simulink model "tesdd"  (R2012b)
(part 2 of 52)

      | %     current_names = textscan(strtrim(strrep(strrep(get_param(blk, 'names'), ']', ''), '[', '')), '%s');
      | %     current_names = current_names{1};
      | %     numios = length(current_names);
      | %     if length(current_types) ~= numios,
      | %         error('%d field names specified, but %d types?', numios, length(current_types));
      | %     end
      | % end
      | problem = 0;
      | for ctr = 1 : numios,
      |     t = current_types(ctr);
      |     if (t < 0) || (t > 2),
      |         problem = t;
      |         ctr = numios + 1;
      |     end
      | end
      | if problem ~= 0,
      |     error('Type cannot be %i, must be 0, 1 or 2.', problem);
      | end
      mask Callback bin_pts:
      | swreg_maskcheck(gcb);
      | % blk = gcb;
      | % mode = get_param(blk, 'mode');
      | % current_bins = eval(get_param(blk, 'bin_pts'));
      | % if (strcmp(mode, 'one value') || strcmp(mode, 'fields of equal size')) && (length(current_bins) > 1),
      | %     error('Only one binary pt may be specified for this mode.');
      | % elseif strcmp(mode, 'fields of arbitrary size')
      | %     current_names = textscan(strtrim(strrep(strrep(get_param(blk, 'names'), ']', ''), '[', '')), '%s');
      | %     current_names = current_names{1};
      | %     numios = length(current_names);
      | %     if length(current_bins) ~= numios,
      | %         error('%d field names specified, but %d binary pts?', numios, length(current_bins));
      | %     end
      | % end
  sw_timestamp2 : Subsystem  Tag=xps:sw_reg  AncestorBlock=xps_library/software register  mask(swreg){mode=one value, io_dir=From Processor, io_delay=0, sample_period=1, names=reg, bitwidths=32, arith_types=0, bin_pts=0, sim_port=on, show_format=off}
      mask prompts: io_dir "I/O direction"; io_delay "I/O delay"; sample_period "Sample period"; names "Name:"; bitwidths "Bitwidth:"; arith_types "Type (ufix=0, fix=1, bool=2):"; bin_pts "Binary pt:"; sim_port "Provide sim input/output?"; show_format "Print format string?"
      mask init:
      | swreg_init(gcb)
      settings: AttributesFormatString=1input
      mask TypeOptions mode: one value | fields of equal size | fields of arbitrary size
      mask Callback mode: swreg_cb(gcb);
      mask TypeOptions io_dir: To Processor | From Processor
      mask Callback io_dir:
      | mask_enables = get_param(gcb, 'MaskEnables');
      | mask_names = get_param(gcb, 'MaskNames');
      | if strcmp(get_param(gcb, 'io_dir'), 'To Processor'),
      |     mask_enables{ismember(mask_names, 'sample_period')} = 'off';
      | else
      |     mask_enables{ismember(mask_names, 'sample_period')} = 'on';
      | end
      | set_param(gcb, 'MaskEnables', mask_enables);
      mask Callback bitwidths:
      | swreg_maskcheck(gcb);
      | % blk = gcb;
      | % mode = get_param(blk, 'mode');
      | % current_widths = eval(get_param(blk, 'bitwidths'));
      | % if (strcmp(mode, 'one value') || strcmp(mode, 'fields of equal size')) && (length(current_widths) > 1),
      | %     error('Only one width may be specified for this mode.');
      | % elseif strcmp(mode, 'fields of arbitrary size')
      | %     current_names = textscan(strtrim(strrep(strrep(get_param(blk, 'names'), ']', ''), '[', '')), '%s');
      | %     current_names = current_names{1};
      | %     numios = length(current_names);
      | %     if length(current_widths) ~= numios,
      | %         error('%d field names specified, but %d widths?', numios, length(current_widths));
      | %     end
      | % end
      | % total_width = 0;
      | % for ctr = 1 : length(current_widths),
      | %     total_width = total_width + current_widths(ctr);
      | % end
      | % if total_width > 32,
      | %     error('Total width must be 32 or less, set to %d.', total_width);
      | % end
      mask Callback arith_types:
      | [numios, ~, ~, ~, current_types] = swreg_maskcheck(gcb);
      | % blk = gcb;
      | % mode = get_param(blk, 'mode');
      | % current_types = eval(get_param(blk, 'arith_types'));
      | % numios = length(current_types);
      | % if (strcmp(mode, 'one value') || strcmp(mode, 'fields of equal size')) && (length(current_types) > 1),
      | %     error('Only one type may be specified for this mode.');
      | % elseif strcmp(mode, 'fields of arbitrary size')
      | %     current_names = textscan(strtrim(strrep(strrep(get_param(blk, 'names'), ']', ''), '[', '')), '%s');
      | %     current_names = current_names{1};
      | %     numios = length(current_names);
      | %     if length(current_types) ~= numios,
      | %         error('%d field names specified, but %d types?', numios, length(current_types));
      | %     end
      | % end
      | problem = 0;
      | for ctr = 1 : numios,
      |     t = current_types(ctr);
      |     if (t < 0) || (t > 2),
      |         problem = t;
      |         ctr = numios + 1;
      |     end
      | end
      | if problem ~= 0,
      |     error('Type cannot be %i, must be 0, 1 or 2.', problem);
      | end
      mask Callback bin_pts:
      | swreg_maskcheck(gcb);
      | % blk = gcb;
      | % mode = get_param(blk, 'mode');
      | % current_bins = eval(get_param(blk, 'bin_pts'));
      | % if (strcmp(mode, 'one value') || strcmp(mode, 'fields of equal size')) && (length(current_bins) > 1),
      | %     error('Only one binary pt may be specified for this mode.');
      | % elseif strcmp(mode, 'fields of arbitrary size')
      | %     current_names = textscan(strtrim(strrep(strrep(get_param(blk, 'names'), ']', ''), '[', '')), '%s');
      | %     current_names = current_names{1};
      | %     numios = length(current_names);
      | %     if length(current_bins) ~= numios,
      | %         error('%d field names specified, but %d binary pts?', numios, length(current_bins));
      | %     end
      | % end
  syncDelay : Subsystem  Tag=xps:sw_reg  AncestorBlock=xps_library/software register  mask(swreg){mode=one value, io_dir=From Processor, io_delay=0, sample_period=1, names=reg, bitwidths=16, arith_types=0, bin_pts=0, sim_port=on, show_format=off}
      mask prompts: io_dir "I/O direction"; io_delay "I/O delay"; sample_period "Sample period"; names "Name:"; bitwidths "Bitwidth:"; arith_types "Type (ufix=0, fix=1, bool=2):"; bin_pts "Binary pt:"; sim_port "Provide sim input/output?"; show_format "Print format string?"
      mask init:
      | swreg_init(gcb)
      settings: AttributesFormatString=1input
      mask TypeOptions mode: one value | fields of equal size | fields of arbitrary size
      mask Callback mode: swreg_cb(gcb);
      mask TypeOptions io_dir: To Processor | From Processor
      mask Callback io_dir:
      | mask_enables = get_param(gcb, 'MaskEnables');
      | mask_names = get_param(gcb, 'MaskNames');
      | if strcmp(get_param(gcb, 'io_dir'), 'To Processor'),
      |     mask_enables{ismember(mask_names, 'sample_period')} = 'off';
      | else
      |     mask_enables{ismember(mask_names, 'sample_period')} = 'on';
      | end
      | set_param(gcb, 'MaskEnables', mask_enables);
      mask Callback bitwidths:
      | swreg_maskcheck(gcb);
      | % blk = gcb;
      | % mode = get_param(blk, 'mode');
      | % current_widths = eval(get_param(blk, 'bitwidths'));
      | % if (strcmp(mode, 'one value') || strcmp(mode, 'fields of equal size')) && (length(current_widths) > 1),
      | %     error('Only one width may be specified for this mode.');
      | % elseif strcmp(mode, 'fields of arbitrary size')
      | %     current_names = textscan(strtrim(strrep(strrep(get_param(blk, 'names'), ']', ''), '[', '')), '%s');
      | %     current_names = current_names{1};
      | %     numios = length(current_names);
      | %     if length(current_widths) ~= numios,
      | %         error('%d field names specified, but %d widths?', numios, length(current_widths));
      | %     end
      | % end
      | % total_width = 0;
      | % for ctr = 1 : length(current_widths),
      | %     total_width = total_width + current_widths(ctr);
      | % end
      | % if total_width > 32,
      | %     error('Total width must be 32 or less, set to %d.', total_width);
      | % end
      mask Callback arith_types:
      | [numios, ~, ~, ~, current_types] = swreg_maskcheck(gcb);
      | % blk = gcb;
      | % mode = get_param(blk, 'mode');
      | % current_types = eval(get_param(blk, 'arith_types'));
      | % numios = length(current_types);
      | % if (strcmp(mode, 'one value') || strcmp(mode, 'fields of equal size')) && (length(current_types) > 1),
      | %     error('Only one type may be specified for this mode.');
      | % elseif strcmp(mode, 'fields of arbitrary size')
      | %     current_names = textscan(strtrim(strrep(strrep(get_param(blk, 'names'), ']', ''), '[', '')), '%s');
      | %     current_names = current_names{1};
      | %     numios = length(current_names);
      | %     if length(current_types) ~= numios,
      | %         error('%d field names specified, but %d types?', numios, length(current_types));
      | %     end
      | % end
      | problem = 0;
      | for ctr = 1 : numios,
      |     t = current_types(ctr);
      |     if (t < 0) || (t > 2),
      |         problem = t;
      |         ctr = numios + 1;
      |     end
      | end
      | if problem ~= 0,
      |     error('Type cannot be %i, must be 0, 1 or 2.', problem);
      | end
      mask Callback bin_pts:
      | swreg_maskcheck(gcb);
      | % blk = gcb;
      | % mode = get_param(blk, 'mode');
      | % current_bins = eval(get_param(blk, 'bin_pts'));
      | % if (strcmp(mode, 'one value') || strcmp(mode, 'fields of equal size')) && (length(current_bins) > 1),
      | %     error('Only one binary pt may be specified for this mode.');
      | % elseif strcmp(mode, 'fields of arbitrary size')
      | %     current_names = textscan(strtrim(strrep(strrep(get_param(blk, 'names'), ']', ''), '[', '')), '%s');
      | %     current_names = current_names{1};
      | %     numios = length(current_names);
      | %     if length(current_bins) ~= numios,
      | %         error('%d field names specified, but %d binary pts?', numios, length(current_bins));
      | %     end
      | % end
  sync_bit1 : xbsIndex_r4/Slice  nbits=1  boolean_output=on  mode=Upper Bit Location + Width  bit1=-2  base1=MSB of Input  bit0=0  base0=LSB of Input  dbl_ovrd=off  block_type=slice
  sync_bit7 : xbsIndex_r4/Slice  nbits=1  boolean_output=on  mode=Upper Bit Location + Width  bit1=-2  base1=MSB of Input  bit0=0  base0=LSB of Input  dbl_ovrd=off  block_type=slice
  sync_in : xps_library/gpio  Tag=xps:gpio  io_group=ROACH2:sync_in  io_dir=in  arith_type=Boolean  bitwidth=1  bin_pt=0  bit_index=0  sample_period=1  use_single_ended=off  use_ddr=off  reg_iob=on  reg_clk_phase=0  termination=None
  sync_out : xps_library/gpio  Tag=xps:gpio  io_group=ROACH2:sync_out  io_dir=out  arith_type=Boolean  bitwidth=1  bin_pt=0  bit_index=0  sample_period=1  use_single_ended=off  use_ddr=off  reg_iob=on  reg_clk_phase=0  termination=None
  top16_{1..8} (8 alike) : xbsIndex_r4/Slice  nbits=16  boolean_output=off  mode=Upper Bit Location + Width  bit1=0  base1=MSB of Input  bit0=0  base0=MSB of Input  dbl_ovrd=off  block_type=slice
  txdestip : Subsystem  Tag=xps:sw_reg  AncestorBlock=xps_library/software register  mask(swreg){mode=one value, io_dir=From Processor, io_delay=0, sample_period=1, names=reg, bitwidths=32, arith_types=0, bin_pts=0, sim_port=on, show_format=off}
      mask prompts: io_dir "I/O direction"; io_delay "I/O delay"; sample_period "Sample period"; names "Name:"; bitwidths "Bitwidth:"; arith_types "Type (ufix=0, fix=1, bool=2):"; bin_pts "Binary pt:"; sim_port "Provide sim input/output?"; show_format "Print format string?"
      mask init:
      | swreg_init(gcb)
      settings: AttributesFormatString=1input
      mask TypeOptions mode: one value | fields of equal size | fields of arbitrary size
      mask Callback mode: swreg_cb(gcb);
      mask TypeOptions io_dir: To Processor | From Processor
      mask Callback io_dir:
      | mask_enables = get_param(gcb, 'MaskEnables');
      | mask_names = get_param(gcb, 'MaskNames');
      | if strcmp(get_param(gcb, 'io_dir'), 'To Processor'),
      |     mask_enables{ismember(mask_names, 'sample_period')} = 'off';
      | else
      |     mask_enables{ismember(mask_names, 'sample_period')} = 'on';
      | end
      | set_param(gcb, 'MaskEnables', mask_enables);
      mask Callback bitwidths:
      | swreg_maskcheck(gcb);
      | % blk = gcb;
      | % mode = get_param(blk, 'mode');
      | % current_widths = eval(get_param(blk, 'bitwidths'));
      | % if (strcmp(mode, 'one value') || strcmp(mode, 'fields of equal size')) && (length(current_widths) > 1),
      | %     error('Only one width may be specified for this mode.');
      | % elseif strcmp(mode, 'fields of arbitrary size')
      | %     current_names = textscan(strtrim(strrep(strrep(get_param(blk, 'names'), ']', ''), '[', '')), '%s');
      | %     current_names = current_names{1};
      | %     numios = length(current_names);
      | %     if length(current_widths) ~= numios,
      | %         error('%d field names specified, but %d widths?', numios, length(current_widths));
      | %     end
      | % end
      | % total_width = 0;
      | % for ctr = 1 : length(current_widths),
      | %     total_width = total_width + current_widths(ctr);
      | % end
      | % if total_width > 32,
      | %     error('Total width must be 32 or less, set to %d.', total_width);
      | % end
      mask Callback arith_types:
      | [numios, ~, ~, ~, current_types] = swreg_maskcheck(gcb);
      | % blk = gcb;
      | % mode = get_param(blk, 'mode');
      | % current_types = eval(get_param(blk, 'arith_types'));
      | % numios = length(current_types);
      | % if (strcmp(mode, 'one value') || strcmp(mode, 'fields of equal size')) && (length(current_types) > 1),
      | %     error('Only one type may be specified for this mode.');
      | % elseif strcmp(mode, 'fields of arbitrary size')
      | %     current_names = textscan(strtrim(strrep(strrep(get_param(blk, 'names'), ']', ''), '[', '')), '%s');
      | %     current_names = current_names{1};
      | %     numios = length(current_names);
      | %     if length(current_types) ~= numios,
      | %         error('%d field names specified, but %d types?', numios, length(current_types));
      | %     end
      | % end
      | problem = 0;
      | for ctr = 1 : numios,
      |     t = current_types(ctr);
      |     if (t < 0) || (t > 2),
      |         problem = t;
      |         ctr = numios + 1;
      |     end
      | end
      | if problem ~= 0,
      |     error('Type cannot be %i, must be 0, 1 or 2.', problem);
      | end
      mask Callback bin_pts:
      | swreg_maskcheck(gcb);
      | % blk = gcb;
      | % mode = get_param(blk, 'mode');
      | % current_bins = eval(get_param(blk, 'bin_pts'));
      | % if (strcmp(mode, 'one value') || strcmp(mode, 'fields of equal size')) && (length(current_bins) > 1),
      | %     error('Only one binary pt may be specified for this mode.');
      | % elseif strcmp(mode, 'fields of arbitrary size')
      | %     current_names = textscan(strtrim(strrep(strrep(get_param(blk, 'names'), ']', ''), '[', '')), '%s');
      | %     current_names = current_names{1};
      | %     numios = length(current_names);
      | %     if length(current_bins) ~= numios,
      | %         error('%d field names specified, but %d binary pts?', numios, length(current_bins));
      | %     end
      | % end
  txdestport : Subsystem  Tag=xps:sw_reg  AncestorBlock=xps_library/software register  mask(swreg){mode=one value, io_dir=From Processor, io_delay=0, sample_period=1, names=reg, bitwidths=16, arith_types=0, bin_pts=0, sim_port=on, show_format=off}
      mask prompts: io_dir "I/O direction"; io_delay "I/O delay"; sample_period "Sample period"; names "Name:"; bitwidths "Bitwidth:"; arith_types "Type (ufix=0, fix=1, bool=2):"; bin_pts "Binary pt:"; sim_port "Provide sim input/output?"; show_format "Print format string?"
      mask init:
      | swreg_init(gcb)
      settings: AttributesFormatString=1input
      mask TypeOptions mode: one value | fields of equal size | fields of arbitrary size
      mask Callback mode: swreg_cb(gcb);
      mask TypeOptions io_dir: To Processor | From Processor
      mask Callback io_dir:
      | mask_enables = get_param(gcb, 'MaskEnables');
      | mask_names = get_param(gcb, 'MaskNames');
      | if strcmp(get_param(gcb, 'io_dir'), 'To Processor'),
      |     mask_enables{ismember(mask_names, 'sample_period')} = 'off';
      | else
      |     mask_enables{ismember(mask_names, 'sample_period')} = 'on';
      | end
      | set_param(gcb, 'MaskEnables', mask_enables);
      mask Callback bitwidths:
      | swreg_maskcheck(gcb);
      | % blk = gcb;
      | % mode = get_param(blk, 'mode');
      | % current_widths = eval(get_param(blk, 'bitwidths'));
      | % if (strcmp(mode, 'one value') || strcmp(mode, 'fields of equal size')) && (length(current_widths) > 1),
      | %     error('Only one width may be specified for this mode.');
      | % elseif strcmp(mode, 'fields of arbitrary size')
      | %     current_names = textscan(strtrim(strrep(strrep(get_param(blk, 'names'), ']', ''), '[', '')), '%s');
      | %     current_names = current_names{1};
      | %     numios = length(current_names);
      | %     if length(current_widths) ~= numios,
      | %         error('%d field names specified, but %d widths?', numios, length(current_widths));
      | %     end
      | % end
      | % total_width = 0;
      | % for ctr = 1 : length(current_widths),
      | %     total_width = total_width + current_widths(ctr);
      | % end
      | % if total_width > 32,
      | %     error('Total width must be 32 or less, set to %d.', total_width);
      | % end
      mask Callback arith_types:
      | [numios, ~, ~, ~, current_types] = swreg_maskcheck(gcb);
      | % blk = gcb;
      | % mode = get_param(blk, 'mode');
      | % current_types = eval(get_param(blk, 'arith_types'));
      | % numios = length(current_types);
      | % if (strcmp(mode, 'one value') || strcmp(mode, 'fields of equal size')) && (length(current_types) > 1),
      | %     error('Only one type may be specified for this mode.');
      | % elseif strcmp(mode, 'fields of arbitrary size')
      | %     current_names = textscan(strtrim(strrep(strrep(get_param(blk, 'names'), ']', ''), '[', '')), '%s');
      | %     current_names = current_names{1};
      | %     numios = length(current_names);
      | %     if length(current_types) ~= numios,
      | %         error('%d field names specified, but %d types?', numios, length(current_types));
      | %     end
      | % end
      | problem = 0;
      | for ctr = 1 : numios,
      |     t = current_types(ctr);
      |     if (t < 0) || (t > 2),
      |         problem = t;
      |         ctr = numios + 1;
      |     end
      | end
      | if problem ~= 0,
      |     error('Type cannot be %i, must be 0, 1 or 2.', problem);
      | end
      mask Callback bin_pts:
      | swreg_maskcheck(gcb);
      | % blk = gcb;
      | % mode = get_param(blk, 'mode');
      | % current_bins = eval(get_param(blk, 'bin_pts'));
      | % if (strcmp(mode, 'one value') || strcmp(mode, 'fields of equal size')) && (length(current_bins) > 1),
      | %     error('Only one binary pt may be specified for this mode.');
      | % elseif strcmp(mode, 'fields of arbitrary size')
      | %     current_names = textscan(strtrim(strrep(strrep(get_param(blk, 'names'), ']', ''), '[', '')), '%s');
      | %     current_names = current_names{1};
      | %     numios = length(current_names);
      | %     if length(current_bins) ~= numios,
      | %         error('%d field names specified, but %d binary pts?', numios, length(current_bins));
      | %     end
      | % end
  zero_bool_{1..4} (4 alike) : xbsIndex_r4/Constant  const=1  gui_display_data_type=Boolean  arith_type=Boolean  n_bits=36  bin_pt=0  preci_type=Single  exp_width=8  frac_width=24  explicit_period=on  period=1  equ=P=C  opselect=C  inp2=PCIN>>17  opr=+  inp1=P  carry=CIN  dbl_ovrd=off  block_type=constant
  zero_bool_7 : xbsIndex_r4/Constant  const=0  gui_display_data_type=Boolean  arith_type=Boolean  n_bits=36  bin_pt=0  preci_type=Single  exp_width=8  frac_width=24  explicit_period=on  period=1  equ=P=C  opselect=C  inp2=PCIN>>17  opr=+  inp1=P  carry=CIN  dbl_ovrd=off  block_type=constant
  wires:
  SRAM_LUT/9(syncout) -> Delay30/1
  MKID_ADC/9(sync) -> Delay29/1
  bool/1 -> octoscope/11(tr2), octoscope/12(tr3), octoscope/16(we3), octoscope/13(we0), octoscope/15(we2), octoscope/14(we1)
  SRAM_LUT/10(bus128) -> Delay36/1, Delay8/1
  Delay25/1 -> WindowAndFFT/6(In6), octoscope/5(in5)
  Delay21/1 -> WindowAndFFT/4(In4), octoscope/1(In1)
  Delay22/1 -> WindowAndFFT/5(In5), octoscope/2(In2)
  Delay26/1 -> octoscope/6(in6), WindowAndFFT/8(In8)
  Delay23/1 -> octoscope/3(In3), WindowAndFFT/7(In7)
  Delay27/1 -> WindowAndFFT/9(In9), octoscope/7(in7)
  Delay24/1 -> octoscope/4(In4), WindowAndFFT/11(In11)
  Delay28/1 -> WindowAndFFT/10(In10), octoscope/8(in8)
  zero_bool_3/1 -> FIFO64_4/7, FIFO64_4/8
  FIFO64_4/8 -> Delay59/1
  [rdchan_a] -> FIFO64_4/4
  fifoRdSettingsA/1(Out1) -> [dumpfifo]
  fifoRdSettingsA/3(Out3) -> [wrrawdata]
  fifoRdSettingsA/4(Out4) -> [is_look_sync]
  fifoRdSettingsA/5(Out5) -> [flushfifo]
  Constant/1 -> lastReadChanA/1(sim_1)
  fifoRdSettingsA/6(Out6) -> [fiforst]
  [fiforst] -> FIFO64_4/6
  [fiford1] -> FIFO64_4/5
  extract_sync_enable_2/2(cmplx_dout) -> dataformatter2/3(data)
  [rdchan_b] -> FIFO64_2/4
  [fiford2] -> FIFO64_2/5
  [fiforst] -> FIFO64_2/6
  FIFO64_2/1 -> extract_sync_enable_2/2(cmplx_din)
  FIFO64_2/8 -> Delay20/1
  fftcoefselector/11(fftfoecsync) -> Delay35/1, [fft_coef_sync]
  zero_bool_7/1 -> octoscope1/15(we2), octoscope1/14(we1), octoscope1/13(we0), octoscope1/12(tr3), octoscope1/10(tr1), octoscope1/11(tr2), octoscope1/16(we3)
  fifoRdSettingsA/7(Out7) -> [drop_all_events]
  fifoRdSettingsA/8(Out8) -> [ethernet_rst]
  [fiforst] -> FIFO64_1/6
  [fiforst] -> FIFO64_3/6
  [dumpfifo] -> MCode2/1
  FIFO64_3/2 -> MCode2/2
  FIFO64_3/5 -> MCode2/3
  FIFO64_3/8 -> Delay6/1
  [rdchan_b] -> FIFO64_3/4
  [rdchan_a] -> FIFO64_1/4
  [fiford1] -> FIFO64_1/5
  [fiford2] -> FIFO64_3/5
  dataformatter1/1(dout) -> Delay15/1
  Delay8/1 -> MKID_DAC/1(buss128)
  Delay29/1 -> octoscope/9(tr0)
  Delay30/1 -> fftcoefselector/2(lut_sync), octoscope/10(tr1)
  fifoRdSettingsA/9(Out9) -> [rst_full_counters]
  Counter3/1 -> fifowriB/1(out_reg)
  [rst_full_counters] -> Counter3/1
  Counter4/1 -> fifowrC/1(out_reg)
  [rst_full_counters] -> Counter4/1
  Counter5/1 -> fifowrD/1(out_reg)
  [rst_full_counters] -> Counter21/1
  Counter7/1 -> evtfifowrB/1(out_reg)
  [rst_full_counters] -> Counter7/1
  Counter9/1 -> outfifowrB/1(out_reg)
  [rst_full_counters] -> Counter9/1
  [datapath_enableb] -> extract_sync_enable_2/4(en)
  Delay20/1 -> extract_sync_enable_2/1(dvld_in)
  [datapath_enableb] -> extract_sync_enable_1/4(en)
  extract_sync_enable_1/2(cmplx_dout) -> dataformatter1/3(data)
  c_to_ri3/1 -> top16_8/1
  c_to_ri4/1 -> top16_2/1
  c_to_ri1/1 -> top16_3/1
  c_to_ri3/2 -> top16_5/1
  c_to_ri4/2 -> top16_6/1
  c_to_ri1/2 -> top16_7/1
  Delay35/1 -> octoscope1/9(tr0)
  Delay31/1 -> c_to_ri2/1
  Delay32/1 -> c_to_ri3/1
  Delay33/1 -> c_to_ri4/1
  Delay34/1 -> c_to_ri1/1
  top16_2/1 -> octoscope1/3(In3)
  top16_3/1 -> octoscope1/4(In4)
  top16_4/1 -> octoscope1/5(in5)
  top16_5/1 -> octoscope1/6(in6)
  top16_6/1 -> octoscope1/7(in7)
  top16_7/1 -> octoscope1/8(in8)
  Delay36/1 -> MKID_ADC/1(in128)
  fftcoefselector/13(topfbsyncin) -> WindowAndFFT/2(In2), [start_fft_sync]
  c_to_ri2/1 -> top16_1/1
  c_to_ri2/2 -> top16_4/1
  top16_1/1 -> octoscope1/1(In1)
  top16_8/1 -> octoscope1/2(In2)
  Concat/1 -> FIFO64_3/3
  Concat4/1 -> FIFO64_1/3
  Concat2/1 -> FIFO64_2/3
  Concat3/1 -> FIFO64_4/3
  [is_look_sync] -> dataformatter1/4(is_pulse)
  [is_look_sync] -> dataformatter2/4(is_pulse)
  Constant5/1 -> syncDelay/1(sim_1)
  Pulse Generator/1 -> sync_in/1
  fifoRdSettingsA/2(Out2) -> [fsmrst]
  lastReadChanA/1(in_reg) -> Delay3/1
  Constant6/1 -> readFifoSize/1(sim_1)
  [fsmrst] -> MCode2/4
  MCode2/3 -> lsb0_5_1/1, [current_chan2]
  MCode2/5 -> [datapath_enableb]
  extract_sync_enable_1/1(dvld_out) -> MCode2/5
  [flushfifo] -> MCode2/8
  [is_look_sync] -> MCode2/11
  bool_5/1 -> MCode2/7
  bool_6/1 -> MCode2/12
  sync_bit1/1 -> Delay43/1
  Delay43/1 -> MCode2/10
  dataformatter2/1(dout) -> Delay/1
  sync_in/1 -> Delay13/1
  fifoRdSettingsA/10(Out10) -> [sync_source]
  [sync_source] -> Mux/1
  RampGenerator/1(ramp) -> SigmaDeltaSecOrder/1(DataIn)
  RampGenerator/2(syncout) -> Mux/3
  Constant2/1 -> sw_timestamp2/1(sim_1)
  fftcoefselector/17(timestamp) -> [fftcounter]
  extract_sync_enable_2/4(swts) -> [swtimestamp2bit_1]
  sw_timestamp/1(in_reg) -> Delay1/1
  FIFO64_3/1 -> sync_bit1/1, extract_sync_enable_1/2(cmplx_din)
  Counter14/1 -> numdoneevts1/1(out_reg)
  [rst_full_counters] -> Counter14/1
  Counter19/1 -> evtfifordB/1(out_reg)
  [rst_full_counters] -> Counter19/1
  Constant3/1 -> sw_timestamp/1(sim_1)
  SigmaDeltaSecOrder/1(DataOut) -> Delay4/1
  Delay4/1 -> Delay12/1
  fifoRdSettingsA/11(Out11) -> [en_ramp_gen]
  [en_ramp_gen] -> Delay4/2
  MCode2/6 -> [wr_data_sel2]
  MCode2/2 -> [wr_big_fifo2], Counter7/2
  fifoRdSettingsA/12(Out12) -> [fluxdemod]
  fifoRdSettingsA/13(Out13) -> [savefluxraw]
  [fsmrst] -> Delay38/1
  [flushfifo] -> Delay39/1
  FRD1/1(evt_fifo_rd) -> datacombine/8(rddata), Counter19/2
  [fluxdemod] -> Delay40/1
  [savefluxraw] -> Delay42/1
  FRD1/3(out_wr) -> Delay46/1, Counter9/2
  Counter20/1 -> chanFifoFull2/1(out_reg)
  FIFO64_1/6 -> Counter20/2
  [rst_full_counters] -> Counter20/1
  Counter21/1 -> chanFifoFull3/1(out_reg)
  FIFO64_3/6 -> Counter21/2
  [savetranslated] -> Delay41/1
  RampTimingNew/1(synctofft) -> [syncsave]
  [rst_full_counters] -> RampTimingNew/1(rstcnt)
  sw_timestamp2/1(in_reg) -> Delay7/1
  [fft_coef_sync] -> RampTimingNew/3(fftcoefsync)
  syncDelay/1(in_reg) -> Delay9/1
  Mux/1 -> edge_detect/1(in), RampTimingNew/5(sync)
  RampTimingNew/2(numsync1) -> Delay10/1
  RampTimingNew/3(numsync) -> Delay11/1
  fftcoefselector/12(fftshiftx) -> WindowAndFFT/1(In1)
  fftcoefselector/15(stopfft) -> WindowAndFFT/3(In3)
  WindowAndFFT/2(fft2dly) -> FM/9(fft2dky), Delay31/1
  WindowAndFFT/4(fft2) -> FM/11(fft2), Delay33/1
  WindowAndFFT/5(fft3) -> FM/12(fft3), Delay34/1
  WindowAndFFT/1(Out5) -> fftcoefselector/1(fftsyncout)
  WindowAndFFT/3(fft3dly) -> FM/10(fft3dly), Delay32/1
  FM/9(dvldout4) -> FIFO64_3/2, Counter5/2
  FM/12(dout4) -> Concat/2
  FM/10(dout3) -> Concat4/2
  FM/6(dout2) -> Concat2/2
  FM/3(dout1) -> Concat3/2
  fftcoefselector/4(we2) -> FM/1(ff2d_dval), FM/3(f2_dval)
  fftcoefselector/5(we3) -> FM/2(f3d_dval), FM/4(f3dval)
  fftcoefselector/8(chan2) -> FM/5(f2dchan), FM/7(f2chan)
  fftcoefselector/9(chan3) -> FM/6(f3dchan), FM/8(f3chan)
  [start_fft_sync] -> FM/13(rstaccum)
  FM/8(chanout3) -> FIFO64_1/1
  FM/11(chanout4) -> FIFO64_3/1
  FIFO64_2/4 -> Terminator5/1
  FIFO64_2/5 -> Terminator6/1
  FIFO64_2/6 -> Terminator7/1
  FIFO64_2/7 -> Terminator8/1
  FIFO64_2/9 -> Terminator9/1
  FIFO64_4/4 -> Terminator/1
  FIFO64_4/5 -> Terminator1/1
  FIFO64_4/6 -> Terminator2/1
  FIFO64_4/7 -> Terminator3/1
  FIFO64_4/9 -> Terminator4/1
  zero_bool_1/1 -> FIFO64_2/8, FIFO64_2/7
  zero_bool_2/1 -> FIFO64_1/8, FIFO64_1/7
  zero_bool_4/1 -> FIFO64_3/7, FIFO64_3/8
  Counter2/1 -> fifowrA/1(out_reg)
  fifoRdSettingsA/14(Out14) -> [savetranslated]
  [rst_full_counters] -> Counter2/1
  [syncsave] -> Concat/1
  [syncsave] -> Concat4/1
  [syncsave] -> Concat2/1
  [syncsave] -> Concat3/1
  [rst_full_counters] -> Counter5/1
  [event_length] -> MCode2/9
  readFifoSize/1(in_reg) -> Delay2/1
  [last_channel] -> MCode2/6
  [current_chan2] -> extract_sync_enable_2/3(chan)
  [current_chan2] -> dataformatter2/2(channel_)
  [wr_big_fifo2] -> Delay14/1
  [wr_data_sel2] -> dataformatter2/5(wr_data_sel)
  [swtimestamp32] -> dataformatter2/1(timestamp32_)
  [swtimestamp32] -> dataformatter1/1(timestamp32_)
  [current_chan2] -> extract_sync_enable_1/3(chan)
  [current_chan2] -> dataformatter1/2(channel_)
  MCode2/1 -> [fiford2]
  [wr_data_sel2] -> dataformatter1/5(wr_data_sel)
  [wr_big_fifo2] -> Delay16/1
  [ethernet_rst] -> Delay48/1
  [fsmrst] -> Delay49/1
  [flushfifo] -> Delay50/1
  txdestip/1(in_reg) -> Delay51/1
  txdestport/1(in_reg) -> Delay52/1
  [rst_full_counters] -> Delay47/1
  FRD1/2(dataout) -> Delay45/1
  GBEthernet/1(numtxeof) -> gbeofcount/1(out_reg)
  GBEthernet/3(numtxovf) -> gbtxovfcnt/1(out_reg)
  GBEthernet/6(numtxvld) -> gbdatalen/1(out_reg)
  GBEthernet/7(numfiford) -> outfifordA/1(out_reg)
  GBEthernet/10(numrd2) -> outfifordB/1(out_reg)
  Constant1/1 -> txdestport/1(sim_1), txdestip/1(sim_1)
  [event_length] -> Delay44/1
  MultByTwoUI8_/1(Out1) -> FRD1/1(evtlen)
  [event_length] -> Delay17/1
  datacombine/1(evt_fifo_rd) -> SinglaEvtFIFO1/3, SinglaEvtFIFO2/3
  [flushfifo] -> Delay18/1
  [fsmrst] -> Delay19/1
  [save_event2] -> Delay37/1
  SinglaEvtFIFO2/1 -> datacombine/3(data_in)
  SinglaEvtFIFO2/2 -> datacombine/2(fifo_empty)
  datacombine/3(dataout) -> FRD1/3(data_in)
  datacombine/4(empty) -> FRD1/2(fifo_empty)
  datacombine/2(evtdone) -> FRD1/4(new_evt_rdy)
  SinglaEvtFIFO1/1 -> datacombine/7(datain2)
  FM/7(dvldout3) -> FIFO64_1/2, Counter4/2
  MCode2/7 -> [save_event2], Counter14/2
  FM/2(dvalout1) -> FIFO64_4/2, Counter2/2
  FM/1(chanout1) -> FIFO64_4/1
  FM/4(chanout2) -> FIFO64_2/1
  FM/5(dvalout2) -> Counter3/2, FIFO64_2/2
  Delay1/1 -> [swtimestamp32]
  Delay2/1 -> [event_length]
  Delay3/1 -> [last_channel]
  Delay7/1 -> RampTimingNew/2(swts2)
  Delay9/1 -> RampTimingNew/4(syncdelay)
  Delay10/1 -> numSyncPulses1/1(out_reg)
  Delay11/1 -> numSyncPulses/1(out_reg)
  Delay12/1 -> sync_out/1
  Delay13/1 -> Mux/2
  MKID_ADC/1(i0) -> Delay21/1
  MKID_ADC/2(i1) -> Delay22/1
  MKID_ADC/3(i2) -> Delay23/1
  MKID_ADC/4(i3) -> Delay24/1
  MKID_ADC/5(q0) -> Delay25/1
  MKID_ADC/6(q1) -> Delay26/1
  MKID_ADC/7(q2) -> Delay27/1
  MKID_ADC/8(q3) -> Delay28/1
  Delay/1 -> SinglaEvtFIFO1/1
  Delay14/1 -> SinglaEvtFIFO1/2
  Delay15/1 -> SinglaEvtFIFO2/1
  Delay16/1 -> SinglaEvtFIFO2/2
  Delay17/1 -> datacombine/1(evtlen)
  Delay18/1 -> datacombine/6(clr_fifos)
  Delay19/1 -> datacombine/5(rst)
  Delay37/1 -> datacombine/4(new_evt_rdy)
  Delay38/1 -> FRD1/5(rst)
  Delay39/1 -> FRD1/6(clr_fifos)
  Delay40/1 -> FRD1/7(isflux_demod)
  Delay41/1 -> FRD1/9(circletrans)
  Delay42/1 -> FRD1/8(savefluxraw)
  Delay44/1 -> MultByTwoUI8_/1(In1)
  Delay45/1 -> GBEthernet/9(din2)
  Delay46/1 -> GBEthernet/10(wr2)
  Delay47/1 -> GBEthernet/8(rst)
  Delay48/1 -> GBEthernet/1(rstgbe)
  Delay49/1 -> GBEthernet/2(rstfsm)
  Delay50/1 -> GBEthernet/3(clrfifo)
  Delay51/1 -> GBEthernet/4(destip)
  Delay52/1 -> GBEthernet/5(destport)
  edge_detect/1(out) -> [rampsyncedge]
  [rampsyncedge] -> fftcoefselector/3(rampsync)
  [rst_full_counters] -> Counter1/1
  Counter1/1 -> SEFull/1(out_reg)
  SinglaEvtFIFO1/3 -> Counter1/2
  [rst_full_counters] -> Counter6/1
  Counter6/1 -> SEFull1/1(out_reg)
  SinglaEvtFIFO2/3 -> Counter6/2
  [rst_full_counters] -> datacombine/9(rstfull)
  Counter8/1 -> gbfull1/1(out_reg)
  [rst_full_counters] -> Counter10/1, Counter8/1
  GBEthernet/5(full1) -> Counter8/2
  Counter10/1 -> gbfull2/1(out_reg)
  GBEthernet/9(full2) -> Counter10/2
  [rst_full_counters] -> FRD1/10(rstfull)
  Delay6/1 -> extract_sync_enable_1/1(dvld_in)
  extract_sync_enable_4/2(cmplx_dout) -> dataformatter4/3(data)
  [dumpfifo] -> MCode1/1
  dataformatter3/1(dout) -> Delay54/1
  Counter16/1 -> evtfifowrB1/1(out_reg)
  [rst_full_counters] -> Counter16/1
  Counter17/1 -> outfifowrB1/1(out_reg)
  [rst_full_counters] -> Counter17/1
  [datapath_enablea] -> extract_sync_enable_4/4(en)
  Delay59/1 -> extract_sync_enable_4/1(dvld_in)
  [datapath_enablea] -> extract_sync_enable_3/4(en)
  extract_sync_enable_3/2(cmplx_dout) -> dataformatter3/3(data)
  [is_look_sync] -> dataformatter3/4(is_pulse)
  [is_look_sync] -> dataformatter4/4(is_pulse)
  [fsmrst] -> MCode1/4
  MCode1/3 -> lsb0_5_2/1, [current_chan1]
  MCode1/5 -> [datapath_enablea]
  extract_sync_enable_3/1(dvld_out) -> MCode1/5
  [flushfifo] -> MCode1/8
  [is_look_sync] -> MCode1/11
  bool_2/1 -> MCode1/7
  bool_3/1 -> MCode1/12
  sync_bit7/1 -> Delay66/1
  Delay66/1 -> MCode1/10
  dataformatter4/1(dout) -> Delay5/1
  extract_sync_enable_4/4(swts) -> [swtimestamp2bit_2]
  FIFO64_1/1 -> extract_sync_enable_3/2(cmplx_din), sync_bit7/1
  Counter12/1 -> numdoneevts2/1(out_reg)
  [rst_full_counters] -> Counter12/1
  Counter13/1 -> evtfifordB1/1(out_reg)
  [rst_full_counters] -> Counter13/1
  MCode1/6 -> [wr_data_sel1]
  MCode1/2 -> [wr_big_fifo1], Counter16/2
  [fsmrst] -> Delay61/1
  [flushfifo] -> Delay62/1
  FRD2/1(evt_fifo_rd) -> datacombine1/8(rddata), Counter13/2
  [fluxdemod] -> Delay63/1
  [savefluxraw] -> Delay65/1
  FRD2/3(out_wr) -> Delay69/1, Counter17/2
  [savetranslated] -> Delay64/1
  [event_length] -> MCode1/9
  [last_channel] -> MCode1/6
  [current_chan1] -> extract_sync_enable_4/3(chan)
  [current_chan1] -> dataformatter4/2(channel_)
  [wr_big_fifo1] -> Delay53/1
  [wr_data_sel1] -> dataformatter4/5(wr_data_sel)
  [swtimestamp32] -> dataformatter4/1(timestamp32_)
  [swtimestamp32] -> dataformatter3/1(timestamp32_)
  [current_chan1] -> extract_sync_enable_3/3(chan)
  [current_chan1] -> dataformatter3/2(channel_)
  MCode1/1 -> [fiford1]
  [wr_data_sel1] -> dataformatter3/5(wr_data_sel)
  [wr_big_fifo1] -> Delay55/1
  FRD2/2(dataout) -> Delay68/1
  [event_length] -> Delay67/1
  MultByTwoUI8_1/1(Out1) -> FRD2/1(evtlen)
  [event_length] -> Delay56/1
  datacombine1/1(evt_fifo_rd) -> SinglaEvtFIFO3/3, SinglaEvtFIFO4/3
  [flushfifo] -> Delay57/1
  [fsmrst] -> Delay58/1
  [save_event1] -> Delay60/1
  SinglaEvtFIFO4/1 -> datacombine1/3(data_in)
  SinglaEvtFIFO4/2 -> datacombine1/2(fifo_empty)
  datacombine1/3(dataout) -> FRD2/3(data_in)
  datacombine1/4(empty) -> FRD2/2(fifo_empty)
  datacombine1/2(evtdone) -> FRD2/4(new_evt_rdy)
  SinglaEvtFIFO3/1 -> datacombine1/7(datain2)
  MCode1/7 -> [save_event1], Counter12/2
  Delay5/1 -> SinglaEvtFIFO3/1
  Delay53/1 -> SinglaEvtFIFO3/2
  Delay54/1 -> SinglaEvtFIFO4/1
  Delay55/1 -> SinglaEvtFIFO4/2
  Delay56/1 -> datacombine1/1(evtlen)
  Delay57/1 -> datacombine1/6(clr_fifos)
  Delay58/1 -> datacombine1/5(rst)
  Delay60/1 -> datacombine1/4(new_evt_rdy)
  Delay61/1 -> FRD2/5(rst)
  Delay62/1 -> FRD2/6(clr_fifos)
  Delay63/1 -> FRD2/7(isflux_demod)
  Delay64/1 -> FRD2/9(circletrans)
  Delay65/1 -> FRD2/8(savefluxraw)
  Delay67/1 -> MultByTwoUI8_1/1(In1)
  [rst_full_counters] -> Counter11/1
  Counter11/1 -> SEFull2/1(out_reg)
  SinglaEvtFIFO3/3 -> Counter11/2
  [rst_full_counters] -> Counter15/1
  Counter15/1 -> SEFull3/1(out_reg)
  SinglaEvtFIFO4/3 -> Counter15/2
  [rst_full_counters] -> datacombine1/9(rstfull)
  [rst_full_counters] -> FRD2/10(rstfull)
  Delay70/1 -> extract_sync_enable_3/1(dvld_in)
  Delay68/1 -> GBEthernet/6(din1)
  Delay69/1 -> GBEthernet/7(wr1)
  FIFO64_4/1 -> extract_sync_enable_4/2(cmplx_din)
  FIFO64_1/2 -> MCode1/2
  FIFO64_1/5 -> MCode1/3
  FIFO64_1/8 -> Delay70/1
  lsb0_5_2/1 -> [rdchan_a]
  lsb0_5_1/1 -> [rdchan_b]
